simulink model "sldemo"  (Simulink 7.4)
settings: Solver=ode45  StartTime=0.0  StopTime=10.0  RelTol=1e-3
undefined symbols (not defined in the file or in its folder): ctrl, g, I, Kf, m, mu, PBmax, Rr, slip, TB, v0
settings Model: Creator=carlj  LastModifiedBy=alex
settings OptimizationCC: InlineParams=on
settings DebuggingCC: StrictBusMsg=ErrorLevel1

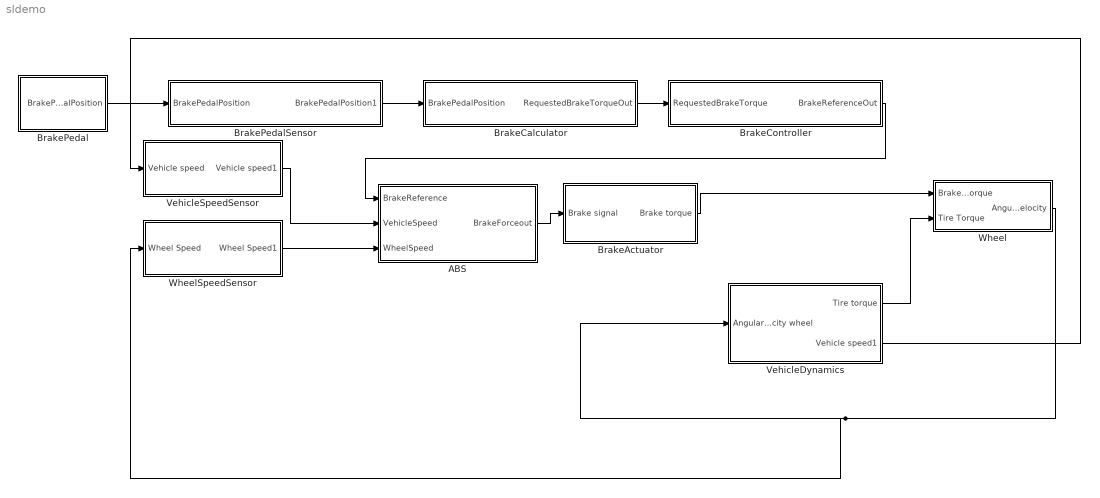
== system sldemo ==
  ABS : Subsystem  TreatAsAtomicUnit=on
  BrakeActuator : Subsystem
  BrakeCalculator : Subsystem
  BrakeController : Subsystem
  BrakePedal : Subsystem
  BrakePedalSensor : Subsystem
  VehicleDynamics : Subsystem
  VehicleSpeedSensor : Subsystem
  Wheel : Subsystem
  "WheelSpeedSensor " : Subsystem
  wires:
  BrakeActuator/1(Brake torque) -> Wheel/1(Brake Torque)
  ABS/1(BrakeForceout) -> BrakeActuator/1(Brake signal)
  Wheel/1(Angular velocity) -> VehicleDynamics/1(Angular velocity wheel), "WheelSpeedSensor "/1(Wheel Speed)
  VehicleSpeedSensor/1(Vehicle speed1) -> ABS/2(VehicleSpeed)
  VehicleDynamics/2(Vehicle speed1) -> VehicleSpeedSensor/1(Vehicle speed)
  VehicleDynamics/1(Tire torque) -> Wheel/2(Tire Torque)
  "WheelSpeedSensor "/1(Wheel Speed1) -> ABS/3(WheelSpeed)
  BrakePedalSensor/1(BrakePedalPosition1) -> BrakeCalculator/1(BrakePedalPosition)
  BrakeCalculator/1(RequestedBrakeTorqueOut) -> BrakeController/1(RequestedBrakeTorque)
  BrakeController/1(BrakeReferenceOut) -> ABS/1(BrakeReference)
  BrakePedal/1(BrakePedalPosition) -> BrakePedalSensor/1(BrakePedalPosition)

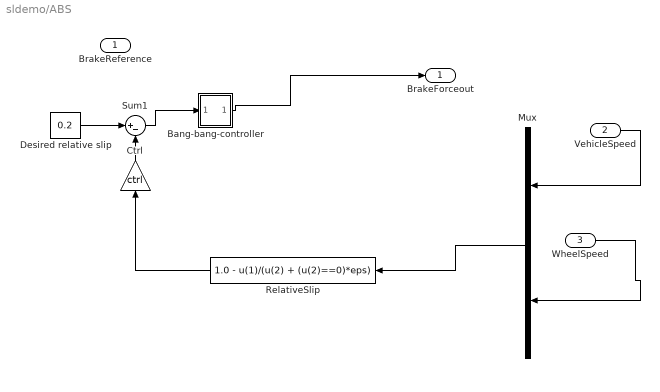
== system sldemo/ABS ==
  BrakeReference : Inport
  VehicleSpeed : Inport  Port=2
  WheelSpeed : Inport  Port=3
  Bang-bang-controller : Subsystem
      mask Type: Sign
      mask Description: y = sign(x)
      mask Help: Sign Function:\n\t\t\ty = 1 if x > 0\n\t\t\ty = 0 if x = 0\n\t\t\ty = -1 if x < 0
      mask Display: plot(-50,-50,50,50,[-50,50],[0,0],[0,0],[-50,50],[-40,0],[-30,-30],[0,40],[30,30])
  Ctrl : Gain  Gain=ctrl  ParameterDataType=sfix(16)  ParameterScaling=2^0  OutDataType=sfix(16)  OutScaling=2^0  SaturateOnIntegerOverflow=on  OutDataTypeStr=Inherit: Same as input  ParamDataTypeStr=Inherit: Same as input
  Desired relative slip : Constant  Value=0.2  OutDataType=sfix(16)  OutScaling=2^0
  Mux : Mux  Inputs=2
  RelativeSlip : Fcn  Expr=1.0 - u(1)/(u(2) + (u(2)==0)*eps)
  Sum1 : Sum  Inputs=|+-  OutDataType=sfix(16)  OutScaling=2^0  SaturateOnIntegerOverflow=on  InputSameDT=on  OutDataTypeStr=Inherit: Same as first input
  BrakeForceout : Outport
  wires:
  Ctrl/1 -> Sum1/2
  Desired relative slip/1 -> Sum1/1
  Sum1/1 -> Bang-bang-controller/1(in_1)
  Bang-bang-controller/1(out_1) -> BrakeForceout/1
  RelativeSlip/1 -> Ctrl/1
  Mux/1 -> RelativeSlip/1
  VehicleSpeed/1 -> Mux/1
  WheelSpeed/1 -> Mux/2

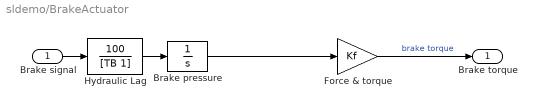
== system sldemo/BrakeActuator ==
  Brake signal : Inport
  Brake pressure : Integrator  LimitOutput=on  UpperSaturationLimit=PBmax  LowerSaturationLimit=0
  Force & torque : Gain  Gain=Kf  ParameterDataType=sfix(16)  ParameterScaling=2^0  OutDataType=sfix(16)  OutScaling=2^0  SaturateOnIntegerOverflow=on  OutDataTypeStr=Inherit: Same as input  ParamDataTypeStr=Inherit: Same as input
  "Hydraulic Lag " : TransferFcn  Numerator=[100]  Denominator=[TB 1]
  Brake torque : Outport
  wires:
  Brake pressure/1 -> Force & torque/1
  "Hydraulic Lag "/1 -> Brake pressure/1
  Force & torque/1 -> Brake torque/1  "brake torque"
  Brake signal/1 -> "Hydraulic Lag "/1

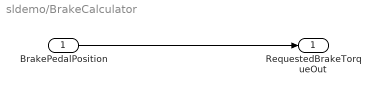
== system sldemo/BrakeCalculator ==
  BrakePedalPosition : Inport  OutDataType=sfix(16)  OutScaling=2^0
  RequestedBrakeTorqueOut : Outport  OutDataType=sfix(16)  OutScaling=2^0
  wires:
  BrakePedalPosition/1 -> RequestedBrakeTorqueOut/1

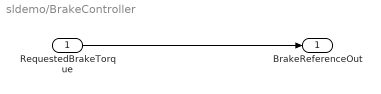
== system sldemo/BrakeController ==
  RequestedBrakeTorque : Inport  OutDataType=sfix(16)  OutScaling=2^0
  BrakeReferenceOut : Outport  OutDataType=sfix(16)  OutScaling=2^0
  wires:
  RequestedBrakeTorque/1 -> BrakeReferenceOut/1

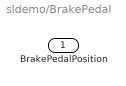
== system sldemo/BrakePedal ==
  BrakePedalPosition : Outport  OutDataType=sfix(16)  OutScaling=2^0

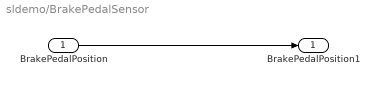
== system sldemo/BrakePedalSensor ==
  BrakePedalPosition : Inport  OutDataType=sfix(16)  OutScaling=2^0
  BrakePedalPosition1 : Outport  OutDataType=sfix(16)  OutScaling=2^0
  wires:
  BrakePedalPosition/1 -> BrakePedalPosition1/1

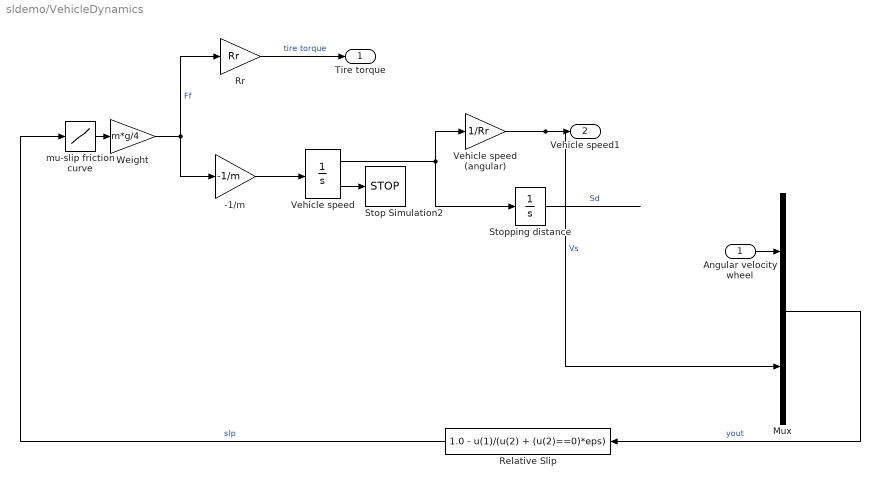
== system sldemo/VehicleDynamics ==
  Angular velocity wheel : Inport
  -1/m : Gain  Gain=-1/m  ParameterDataType=sfix(16)  ParameterScaling=2^0  OutDataType=sfix(16)  OutScaling=2^0  SaturateOnIntegerOverflow=on  OutDataTypeStr=Inherit: Same as input  ParamDataTypeStr=Inherit: Same as input
  Mux : Mux  Inputs=2
  Relative Slip : Fcn  Expr=1.0 - u(1)/(u(2) + (u(2)==0)*eps)
  Rr : Gain  Gain=Rr  ParameterDataType=sfix(16)  ParameterScaling=2^0  OutDataType=sfix(16)  OutScaling=2^0  SaturateOnIntegerOverflow=on  OutDataTypeStr=Inherit: Same as input  ParamDataTypeStr=Inherit: Same as input
  Stop Simulation2 : Stop
  Stopping distance : Integrator  UpperSaturationLimit=1000  LowerSaturationLimit=0
  Vehicle speed : Integrator  InitialCondition=v0  LimitOutput=on  UpperSaturationLimit=1000  LowerSaturationLimit=0  ShowSaturationPort=on
  Vehicle speed (angular) : Gain  Gain=1/Rr  ParameterDataType=sfix(16)  ParameterScaling=2^0  OutDataType=sfix(16)  OutScaling=2^0  SaturateOnIntegerOverflow=on  OutDataTypeStr=Inherit: Same as input  ParamDataTypeStr=Inherit: Same as input
  Weight : Gain  Gain=m*g/4  ParameterDataType=sfix(16)  ParameterScaling=2^0  OutDataType=sfix(16)  OutScaling=2^0  SaturateOnIntegerOverflow=on  OutDataTypeStr=Inherit: Same as input  ParamDataTypeStr=Inherit: Same as input
  mu-slip friction curve : Lookup  InputValues=slip  Table=mu  OutDataType=sfix(16)  OutScaling=2^0  SaturateOnIntegerOverflow=on
  Tire torque : Outport
  Vehicle speed1 : Outport  Port=2
  wires:
  -1/m/1 -> Vehicle speed/1
  Vehicle speed/2 -> Stop Simulation2/1
  Vehicle speed/1 -> Stopping distance/1, Vehicle speed (angular)/1
  mu-slip friction curve/1 -> Weight/1
  Weight/1 -> -1/m/1, Rr/1  "Ff"
  Rr/1 -> Tire torque/1  "tire torque"
  Vehicle speed (angular)/1 -> Vehicle speed1/1, Mux/2  "Vs"
  Stopping distance/1 -> ?  "Sd"
  Mux/1 -> Relative Slip/1  "yout"
  Angular velocity wheel/1 -> Mux/1
  Relative Slip/1 -> mu-slip friction curve/1  "slp"

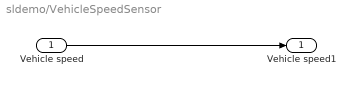
== system sldemo/VehicleSpeedSensor ==
  Vehicle speed : Inport  OutDataType=sfix(16)  OutScaling=2^0
  Vehicle speed1 : Outport  OutDataType=sfix(16)  OutScaling=2^0
  wires:
  Vehicle speed/1 -> Vehicle speed1/1

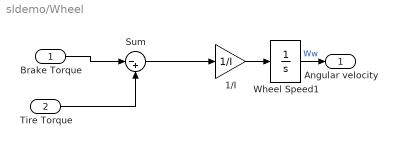
== system sldemo/Wheel ==
  Brake Torque : Inport
  Tire Torque : Inport  Port=2
  1/I : Gain  Gain=1/I  ParameterDataType=sfix(16)  ParameterScaling=2^0  OutDataType=sfix(16)  OutScaling=2^0  SaturateOnIntegerOverflow=on  OutDataTypeStr=Inherit: Same as input  ParamDataTypeStr=Inherit: Same as input
  Sum : Sum  Inputs=|-+  OutDataType=sfix(16)  OutScaling=2^0  SaturateOnIntegerOverflow=on  InputSameDT=on  OutDataTypeStr=Inherit: Same as first input
  Wheel Speed1 : Integrator  InitialCondition=v0/Rr  LimitOutput=on  UpperSaturationLimit=1000  LowerSaturationLimit=0
  Angular velocity : Outport
  wires:
  1/I/1 -> Wheel Speed1/1
  Wheel Speed1/1 -> Angular velocity/1  "Ww"
  Brake Torque/1 -> Sum/1
  Sum/1 -> 1/I/1
  Tire Torque/1 -> Sum/2

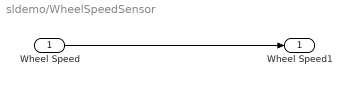
== system sldemo/WheelSpeedSensor  ==
  Wheel Speed : Inport  OutDataType=sfix(16)  OutScaling=2^0
  Wheel Speed1 : Outport  OutDataType=sfix(16)  OutScaling=2^0
  wires:
  Wheel Speed/1 -> Wheel Speed1/1

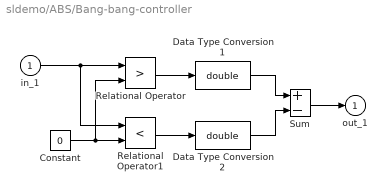
== system sldemo/ABS/Bang-bang-controller ==
  in_1 : Inport  OutDataType=sfix(16)  OutScaling=2^0
  Constant : Constant  Value=0  OutDataType=sfix(16)  OutScaling=2^0
  Data Type Conversion1 : DataTypeConversion  OutDataTypeMode=double  OutDataType=sfix(16)  OutScaling=2^0  OutDataTypeStr=double  SaturateOnIntegerOverflow=on  RndMeth=Zero
  Data Type Conversion2 : DataTypeConversion  OutDataTypeMode=double  OutDataType=sfix(16)  OutScaling=2^0  OutDataTypeStr=double  SaturateOnIntegerOverflow=on  RndMeth=Zero
  Relational Operator : RelationalOperator  Operator=>  InputSameDT=on
  Relational Operator1 : RelationalOperator  Operator=<  InputSameDT=on
  Sum : Sum  Inputs=+-  OutDataType=sfix(16)  OutScaling=2^0  SaturateOnIntegerOverflow=on  InputSameDT=on  OutDataTypeStr=Inherit: Same as first input
  out_1 : Outport  OutDataType=sfix(16)  OutScaling=2^0  InitialOutput=0
  wires:
  Data Type Conversion2/1 -> Sum/2
  Data Type Conversion1/1 -> Sum/1
  Sum/1 -> out_1/1
  Relational Operator/1 -> Data Type Conversion1/1
  Relational Operator1/1 -> Data Type Conversion2/1
  Constant/1 -> Relational Operator/2, Relational Operator1/2
  in_1/1 -> Relational Operator1/1, Relational Operator/1
